simulink model "ROPOD_4Wheel_TdistZMPC_cntr"  (R2017b)
settings: Solver=FixedStepAuto  StartTime=0.0  StopTime=Inf  FixedStep=Ts  RelTol=1e-3
PreLoadFcn:
  | cd /home/robocup/RoPod/Force_dist_ZMPC_ROS
  | init_model
InitFcn:
  | cd /home/robocup/RoPod/Force_dist_ZMPC_ROS
  | init_model
values from neighbouring files (symbols this model uses):
  b_cx = 36.5    [RoPod_parameters.mat]
  b_cy = 36.5    [RoPod_parameters.mat]
  Fd_max = 70    [RoPod_parameters.mat]
  Fd_min = 20    [RoPod_parameters.mat]
  FFtheta_intia = 0    [init_model.m]
  FFxy_mass = 80    [init_model.m]
  Fr_max = 100    [RoPod_parameters.mat]
  Fr_min = -100    [RoPod_parameters.mat]
  k_cx = 1713    [RoPod_parameters.mat]
  k_cy = 4489    [RoPod_parameters.mat]
  max_hw_tau = 7.0    (= 7)    [init_model.m]
  Nwheels = 4    [init_model.m]
  pivot_offs_sws = [2.21 1.873 2.001 3.508]    [init_model.m]
  SW_COM1_ENABLE1 = hex2dec('0001')    [init_model.m]
  SW_COM1_ENABLE2 = hex2dec('0002')    [init_model.m]
  SW_COM1_MODE_TORQUE = bitshift(hex2dec('0000'),2)    [init_model.m]
  SW_COM1_MODE_VELOCITY = bitshift(hex2dec('0002'),2)    [init_model.m]
  SW_COM1_USE_TS = hex2dec('8000')    [init_model.m]
  sw_tau_2_curr = 1/motor_physical_parameters.torqueconstant.value    [init_model.m]
  Taucompfactor = 2.0    (= 2)    [init_model.m]
  Tinit = 1*Tslot    [init_model.m]
  Ts = 0.001    [init_model.m]
  Ts_MPC = 0.001    [init_model.m]
  Tsp = 1    [init_model.m]
  xA = [1 -1 0 0 0 0 0.0206696424966 -0.0206696424966 0 0 0.0298227588181 -0.0298227588181 ... (4080 elements, 102x40)]    [ZMPCx_parameters.mat]
  xBd_dis = [1.12932348493e-06 0.000225071897401 0 0]    [ZMPCx_parameters.mat]
  xF = [0 0 0 0 0 0 0 0 0 0 0 0 ... (80 elements, 20x4)]    [ZMPCx_parameters.mat]
  xH = [20 0 0 0 0 0 0 0 0 0 0 0 ... (1600 elements, 40x40)]    [ZMPCx_parameters.mat]
  xPhi = [0.995143909015 -0.967809158823 0 0 0.980727027327 -1.91066813489 0 0 0.957042868744 -2.81984596436 0 0 ... (320 elements, 80x4)]    [ZMPCx_parameters.mat]
  xrho = 144000    [ZMPCx_parameters.mat]
  xW = [0 0 -4300 4300 0 0 -4211.12053726 4211.12053726 0 0 -4082.88267435 4082.88267435 ... (328 elements, 82x4)]    [ZMPCx_parameters.mat]
  yA = [1 -1 0 0 0 0 0.0146537039222 -0.0146537039222 0 0 0.0255124036215 -0.0255124036215 ... (4080 elements, 102x40)]    [ZMPCy_parameters.mat]
  yBd_dis = [1.24492522358e-06 0.000248362591603 0 0]    [ZMPCy_parameters.mat]
  yF = [0.00191047141222 0.00156448969707 0.00119761396088 0.000813779538874 0.00041715000072 1.20724055612e-05 -0.00039696993291 -0.000805406662726 -0.00120863105559 -0.00160205155743 -0.00198114365531 -0.00234150147928 ... (80 elements, 20x4)]    [ZMPCy_parameters.mat]
  yH = [2.00000002801 0 2.31602594113e-08 0 1.80085634996e-08 0 1.26053094289e-08 0 7.00898668547e-09 0 1.2808124932e-09 0 ... (1600 elements, 40x40)]    [ZMPCy_parameters.mat]
  yPhi = [0.994411530671 -1.11489967371 0 0 0.977778317439 -2.20691845877 0 0 0.950389393786 -3.2640842851 0 0 ... (320 elements, 80x4)]    [ZMPCy_parameters.mat]
  yrho = 10000    [ZMPCy_parameters.mat]
  yW = [0 0 -4489 4489 0 0 -4423.21952309 4423.21952309 0 0 -4308.69434324 4308.69434324 ... (328 elements, 82x4)]    [ZMPCy_parameters.mat]
undefined symbols (not defined in the file or in its folder): DiscIntNeverNeededParam, Pose, ropod_kinmodel_param, Twist, Wrench
libraries: cstblocks x85, robotlib x60, simulink x41, SOEM_EtherCAT_Lib x5, robotcorelib x1
(part 6 of 6)

== matlab function ROPOD_4Wheel_TdistZMPC_cntr/Non-ROS Ropod Controller/wheel flip compensation/MATLAB Function3 ==
  data: tl input; tl_out output; tr input; ropod_kinmodel_param_vec input size=18; tr_out output; kmax input
function [tl_out,tr_out] = fcn(tl, tr, ropod_kinmodel_param_vec, kmax)

[  rW1_1,rW1_2,rW1_3,rW1_4,rW2_1,rW2_2,rW2_3,rW2_4,...
    s_w,...
    d_w, ...
    CW1_1,CW1_2,CW1_3,CW1_4,CW2_1,CW2_2,CW2_3,CW2_4 ...
    ]= extract_kinmodel_parameters(ropod_kinmodel_param_vec);

Fxi = (tl/rW1_1+tr/rW1_2);
Fyi = (tr/rW1_2-tl/rW1_1)*(d_w/(2*s_w));
theta = atan2(Fyi,Fxi);

Fsize = sqrt(Fxi*Fxi+Fyi*Fyi);
if Fsize> 30
   sc = (1+(kmax-1)*abs(sin(theta)));
else
    sc = 1;
end

tl_out = tl*sc;
tr_out = tr*sc;
